simulink model "Plant_R3"  (R2023a)
settings: Solver=ode45  StartTime=0.0  StopTime=200  RelTol=1e-2  EnableMultiTasking=on
values from neighbouring files (symbols this model uses):
  k2 = 50    [ChemBenchData.m]    (also in dati.m)
  VR2 = 850    [ChemBenchData.m]    (also in dati.m)
  z3b = 0.4666    [ChemBenchData.m]    (also in dati.m)
  z3d = 0.0523    [ChemBenchData.m]    (also in dati.m)
  z3e = 0.0032    [ChemBenchData.m]    (also in dati.m)
  z3f = 0.4666    [ChemBenchData.m]    (also in dati.m)
undefined symbols (not defined in the file or in its folder): R3_portata, R3_stati, xk0_mod
settings Model: Creator=scattolini  LastModifiedBy=laura
settings SolverCC: AlgebraicLoopSolver=TrustRegion
settings DataIOCC: LimitDataPoints=on  SaveFormat=Array  SignalLoggingSaveFormat=ModelDataLogs  ReturnWorkspaceOutputs=off
settings OptimizationCC: BlockReduction=off  DefaultParameterBehavior=Inlined  InlineInvariantSignals=on  BufferReuse=off  ExpressionDepthLimit=2147483647  InitFltsAndDblsToZero=on  LifeSpan=inf
settings DebuggingCC: SaveWithParameterizedLinksMsg=none  UnderspecifiedInitializationDetection=Classic  MergeDetectMultiDrivingBlocksExec=none  SignalResolutionControl=TryResolveAllWithWarning  SolverPrmCheckMsg=warning  MultiTaskDSMMsg=warning  MultiTaskCondExecSysMsg=none  FcnCallInpInsideContextMsg=warning  UnconnectedInputMsg=warning  UnconnectedOutputMsg=warning  UnconnectedLineMsg=warning  StateNameClashWarn=warning  SFUnexpectedBacktrackingDiag=warning  SFNoUnconditionalDefaultTransitionDiag=warning  SFExecutionAtInitializationDiag=none  ArithmeticOperatorsInVariantConditions=warning
settings HardwareCC: ProdBitPerPointer=32  ProdBitPerSizeT=32  ProdBitPerPtrDiffT=32  ProdLargestAtomicFloat=None  ProdIntDivRoundTo=Undefined  ProdEndianess=Unspecified  ProdWordSize=32  ProdHWDeviceType=32-bit Generic
settings ModelReferenceCC: EnableRefExpFcnMdlSchedulingChecks=on  PropagateSignalLabelsOutOfModel=off
settings RTWCC: DLArmComputeVersion=19.05
settings CodeAppCC: StateflowObjectComments=on
settings GRTTargetCC: TargetFcnLib=ansi_tfl_tmw.mat  TargetLangStandard=C89/C90 (ANSI)  CombineOutputUpdateFcns=off  GRTInterface=on
settings ConfigComp: CovMetricSettings=dw  CovSaveCumulativeToWorkspaceVar=on  CovSaveSingleToWorkspaceVar=on

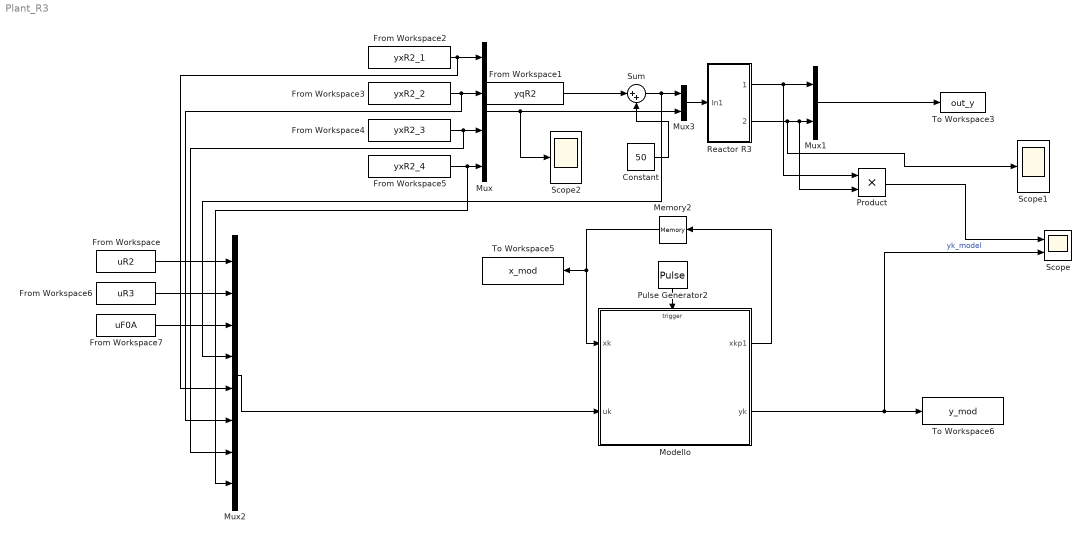
== system Plant_R3 ==
  Constant : Constant  Value=50
  From Workspace : FromWorkspace  VariableName=uR2  SampleTime=-1
  From Workspace1 : FromWorkspace  VariableName=yqR2  SampleTime=-1
  From Workspace2 : FromWorkspace  VariableName=yxR2_1  SampleTime=-1
  From Workspace3 : FromWorkspace  VariableName=yxR2_2  SampleTime=-1
  From Workspace4 : FromWorkspace  VariableName=yxR2_3  SampleTime=-1
  From Workspace5 : FromWorkspace  VariableName=yxR2_4  SampleTime=-1
  From Workspace6 : FromWorkspace  VariableName=uR3  SampleTime=-1
  From Workspace7 : FromWorkspace  VariableName=uF0A  SampleTime=-1
  Memory2 : Memory  InitialCondition=xk0_mod
  "Modello " : Subsystem  TreatAsAtomicUnit=on
  Mux : Mux
  Mux1 : Mux  Inputs=2
  Mux2 : Mux  Inputs=8
  Mux3 : Mux  Inputs=2
  Product : Product
  Pulse Generator2 : DiscretePulseGenerator  PulseType=Time based  Period=1  PulseWidth=5
  Reactor R3 : Subsystem
  Scope : Scope  NumInputPorts=2
  Scope1 : Scope
  Scope2 : Scope
  Sum : Sum  Inputs=|++
  To Workspace3 : ToWorkspace  VariableName=out_y  SampleTime=1
  To Workspace5 : ToWorkspace  VariableName=x_mod  SampleTime=1
  To Workspace6 : ToWorkspace  VariableName=y_mod  SampleTime=1
  wires:
  From Workspace/1 -> Mux2/1
  Mux1/1 -> To Workspace3/1
  From Workspace1/1 -> Sum/1
  Mux/1 -> Scope2/1, Mux3/2
  From Workspace2/1 -> Mux2/5, Mux/1
  From Workspace4/1 -> Mux2/7, Mux/3
  From Workspace5/1 -> Mux2/8, Mux/4
  From Workspace3/1 -> Mux2/6, Mux/2
  "Modello "/1(xkp1) -> Memory2/1
  Memory2/1 -> "Modello "/1(xk), To Workspace5/1
  "Modello "/2(yk) -> Scope/2, To Workspace6/1  "yk_model"
  Pulse Generator2/1 -> "Modello "/Trigger
  Mux2/1 -> "Modello "/2(uk)
  From Workspace6/1 -> Mux2/2
  From Workspace7/1 -> Mux2/3
  Product/1 -> Scope/1
  Mux3/1 -> Reactor R3/1(In1)
  Reactor R3/1(portata) -> Mux1/1, Product/1
  Reactor R3/2(stati B-D-E-F) -> Scope1/1, Product/2, Mux1/2
  Constant/1 -> Sum/2
  Sum/1 -> Mux2/4, Mux3/1

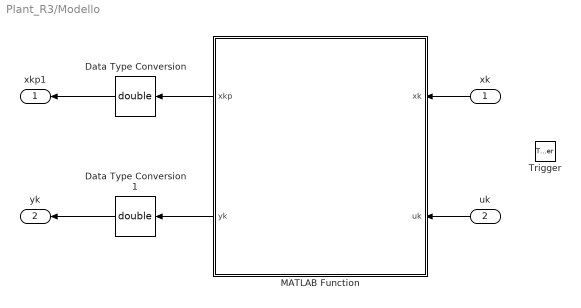
== system Plant_R3/Modello  ==
  xk : Inport
  uk : Inport  Port=2
  Trigger : TriggerPort  VariantControl=(inherit)
  Data Type Conversion : DataTypeConversion  OutDataTypeStr=double  RndMeth=Nearest  SaturateOnIntegerOverflow=off
  Data Type Conversion1 : DataTypeConversion  OutDataTypeStr=double  RndMeth=Nearest  SaturateOnIntegerOverflow=off
  MATLAB Function : MATLAB Function  TreatAsAtomicUnit=on
  xkp1 : Outport
  yk : Outport  Port=2
  wires:
  xk/1 -> MATLAB Function/1(xk)
  MATLAB Function/2(yk) -> Data Type Conversion1/1
  MATLAB Function/1(xkp) -> Data Type Conversion/1
  Data Type Conversion/1 -> xkp1/1
  Data Type Conversion1/1 -> yk/1
  uk/1 -> MATLAB Function/2(uk)

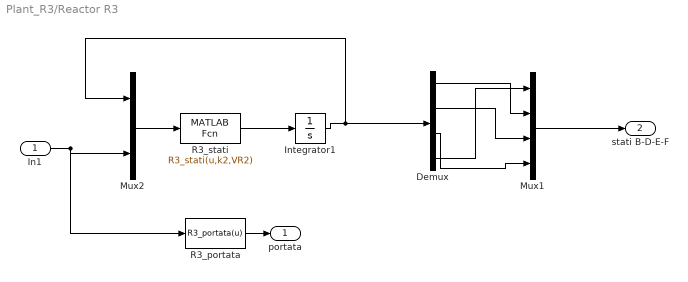
== system Plant_R3/Reactor R3 ==
  In1 : Inport
  Demux : Demux
  Integrator1 : Integrator  InitialCondition=[z3d z3e z3f z3b]
  Mux1 : Mux
  Mux2 : Mux  Inputs=2
  R3_portata : MATLABFcn  MATLABFcn=R3_portata(u)
  R3_stati : MATLABFcn  MATLABFcn=R3_stati(u,k2,VR2)  OutputDimensions=4
  portata : Outport
  stati B-D-E-F : Outport  Port=2
  wires:
  In1/1 -> Mux2/2, R3_portata/1
  R3_stati/1 -> Integrator1/1
  Mux2/1 -> R3_stati/1
  Integrator1/1 -> Mux2/1, Demux/1
  R3_portata/1 -> portata/1
  Demux/4 -> Mux1/1
  Demux/1 -> Mux1/2
  Demux/2 -> Mux1/3
  Demux/3 -> Mux1/4
  Mux1/1 -> stati B-D-E-F/1

== matlab function Plant_R3/Modello /MATLAB Function ==
  data: xkp output; xk input; uk input; yk output
function [xkp, yk] = RNN(xk, uk)

    n_states = [3,3,3,3,3,3];
    layers_file = load("layers_file.mat");
    layers_file = layers_file.layers_file;
    input_scaler_bias = load("input_scaler_bias.mat");
    input_scaler_scale_common = load("input_scaler_scale_common.mat");
    output_scaler_bias = load("output_scaler_bias.mat");
    output_scaler_scale_common = load("output_scaler_scale_common.mat");

    % Scale input and output
    uk3_1 = (uk(1:3)  - (input_scaler_bias.input_scaler_bias(2:4)).') ./ (input_scaler_scale_common.input_scaler_scale_common).';
    uk3_2 = [uk(4)*uk(5); uk(4)*uk(6); uk(4)*uk(7); uk(4)*uk(8)];
    uk3_2 = (uk3_2  - (output_scaler_bias.output_scaler_bias(17:20)).') ./ (output_scaler_scale_common.output_scaler_scale_common).';

     
    % GRU 3
    uk5 = [uk3_1; uk3_2];
    xk5 = xk;
    zk5 = sigmoidfunction((layers_file.layers{1,9}.weights.Wzf(:,1:n_states(5))).' * uk5 + (layers_file.layers{1,9}.weights.Uzf(:,1:n_states(5))).' * xk5 + (layers_file.layers{1,9}.weights.bzf(:,1:n_states(5))).');
    fk5 = sigmoidfunction((layers_file.layers{1,9}.weights.Wzf(:,n_states(5)+1:end)).' * uk5 + (layers_file.layers{1,9}.weights.Uzf(:,n_states(5)+1:end)).' * xk5 + (layers_file.layers{1,9}.weights.bzf(:,n_states(5)+1:end)).');
    phi5 = tanh((layers_file.layers{1,9}.weights.Wr).' * uk5 + (layers_file.layers{1,9}.weights.Ur).' * (fk5.* xk5) + (layers_file.layers{1,9}.weights.br).');
    xkp5 = zk5 .* xk5 + (1-zk5) .* phi5;
    yk5 = layers_file.layers{1,10}.weights.weight * xk5 + (layers_file.layers{1,10}.weights.bias).';

    % Overall
    xkp = xkp5;
    yk = yk5;
    yk = yk .* (output_scaler_scale_common.output_scaler_scale_common).' + (output_scaler_bias.output_scaler_bias(21:24)).';
end
